simulink model "ramp"  (R2015b)
settings: Solver=VariableStepAuto  StartTime=0.0  StopTime=15  RelTol=1e-3
libraries: simulink x1
settings Model: Creator=HP  LastModifiedBy=HP

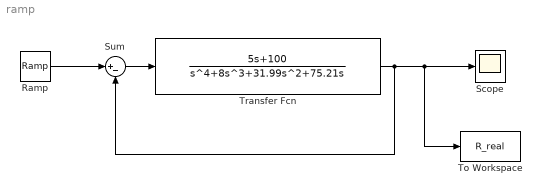
== system ramp ==
  Ramp : simulink/Sources/Ramp  slope=1  start=0  X0=0
  Scope : Scope
  Sum : Sum  Inputs=|+-
  To Workspace : ToWorkspace  VariableName=R_real  SampleTime=0.01
  Transfer Fcn : TransferFcn  Numerator=[0 0 0 5 100]  Denominator=[1 8 31.99 75.21 0]
  wires:
  Sum/1 -> Transfer Fcn/1
  Transfer Fcn/1 -> Sum/2, To Workspace/1, Scope/1
  Ramp/1 -> Sum/1
